simulink subsystem "SensorsRef"  (R2025a)
settings: Solver=VariableStepAuto  StartTime=0.0  StopTime=10.0  RelTol=1e-3
undefined symbols (not defined in the file): Accel_bIb, chi, Euler, gamma, gpsLLA, LaserAlt, Omeg_BIb, Pos_bIi, Q_i2b, SimIn, Vel_bIi, Vtot
libraries: libAxisTransformations x2, starslibMathOperations x2, starslibAxisTransformations x1
settings Model: Creator=drhill  LastModifiedBy=alhallmark
settings SolverCC: AlgebraicLoopSolver=TrustRegion
settings OptimizationCC: ReuseModelBlockBuffer=off
settings DebuggingCC: UnconnectedInputMsg=warning  UnconnectedOutputMsg=warning  UnconnectedLineMsg=warning
settings ModelReferenceCC: EnableRefExpFcnMdlSchedulingChecks=on
settings RTWCC: GPUComputeCapability=3.5  DLArmComputeVersion=19.05

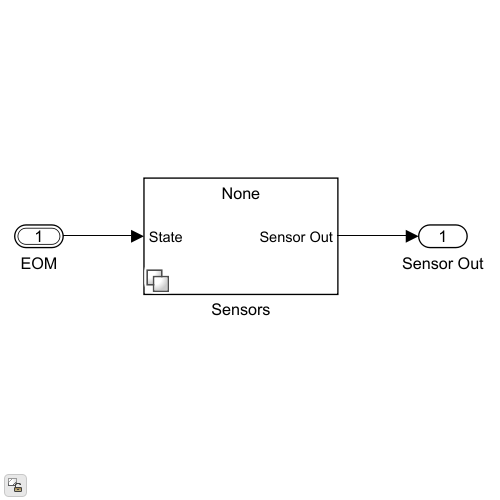
[thumbnail: Simulink's stored preview of the top-level diagram]
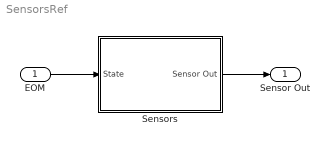
== system SensorsRef ==
  EOM : Inport  OutDataTypeStr=Bus: EomBus
  Sensors : Subsystem  Variant=on
  Sensor Out : Outport
  wires:
  Sensors/1(Sensor Out) -> Sensor Out/1
  EOM/1 -> Sensors/1(State)

== system SensorsRef/Sensors ==
  State : Inport  OutDataTypeStr=Bus: EomBus
  None : Subsystem  VariantControl=GVS_SENSOR_TYPE_NONE
  "ZOH " : Subsystem  VariantControl=GVS_SENSOR_TYPE_ZOH  mask{Sensor=SimIn.Sensor}
      mask prompts: Sensor "Sensor Data"
  Sensor Out : Outport  OutDataTypeStr=Bus: SensorBus  VectorParamsAs1DForOutWhenUnconnected=off

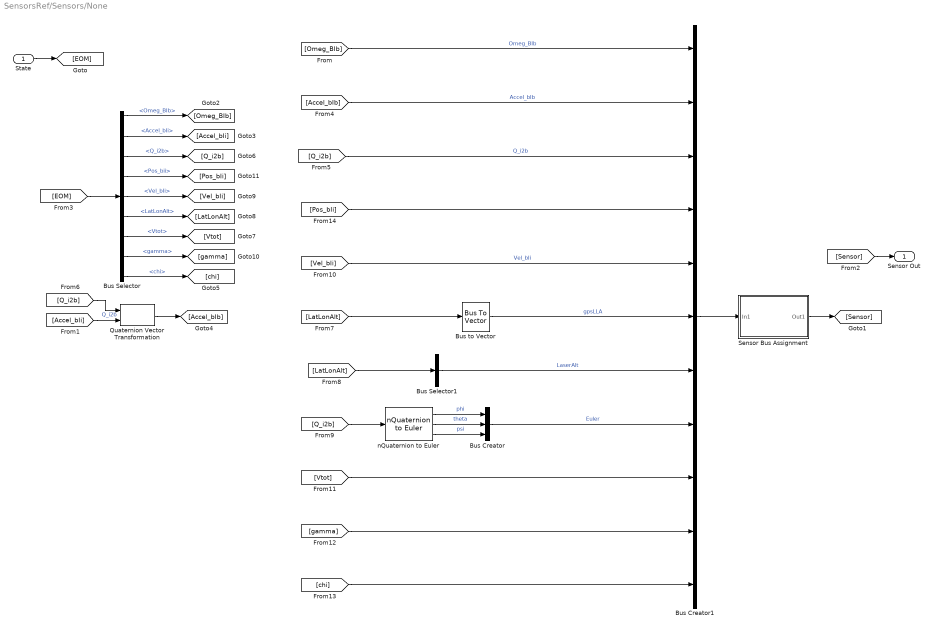
== system SensorsRef/Sensors/None ==
  State : Inport  OutDataTypeStr=Bus: EomBus
  Bus Creator : BusCreator  Inputs=3
  Bus Creator1 : BusCreator  Inputs=11
  Bus Selector : BusSelector  OutputSignals=InertialData.Omeg_BIb,InertialData.Accel_bIi,InertialData.Q_i2b,InertialData.Pos_bii,InertialData.Vel_bIi,WorldRelativeData.LatLonAlt,AirRelativeData.Vtot,AirRelativeData.gamma,AirRelativeData.chi
  Bus Selector1 : BusSelector  OutputSignals=AltGeod  OutputAsBus=on
  Bus to Vector : BusToVector
  Quaternion Vector Transformation : libAxisTransformations/Quaternion Vector Transformation  n=0
  Sensor Bus Assignment : Subsystem
  nQuaternion to Euler : libAxisTransformations/nQuaternion to Euler  n=1  RotOrd=ZYX
  Sensor Out : Outport  OutDataTypeStr=Bus: SensorBus  VectorParamsAs1DForOutWhenUnconnected=off
  wires:
  [Vel_bIi] -> Bus Creator1/5  "Vel_bIi"
  Bus Selector1/1 -> Bus Creator1/7  "LaserAlt"
  [Q_i2b] -> Bus Creator1/3  "Q_i2b"
  [Accel_bIb] -> Bus Creator1/2  "Accel_bIb"
  [Omeg_BIb] -> Bus Creator1/1  "Omeg_BIb"
  Bus Creator1/1 -> Sensor Bus Assignment/1(In1)
  State/1 -> [EOM]
  [EOM] -> Bus Selector/1
  Bus Selector/1 -> [Omeg_BIb]  "<Omeg_BIb>"
  Bus Selector/2 -> [Accel_bIi]  "<Accel_bIi>"
  Bus Selector/3 -> [Q_i2b]  "<Q_i2b>"
  Bus Selector/6 -> [LatLonAlt]  "<LatLonAlt>"
  [LatLonAlt] -> Bus Selector1/1
  Bus Selector/5 -> [Vel_bIi]  "<Vel_bIi>"
  Sensor Bus Assignment/1(Out1) -> [Sensor]
  [Sensor] -> Sensor Out/1
  [Q_i2b] -> Quaternion Vector Transformation/1  "Q_i2b"
  [Accel_bIi] -> Quaternion Vector Transformation/2
  Quaternion Vector Transformation/1 -> [Accel_bIb]
  Bus to Vector/1 -> Bus Creator1/6  "gpsLLA"
  [LatLonAlt] -> Bus to Vector/1
  [Q_i2b] -> nQuaternion to Euler/1
  nQuaternion to Euler/1 -> Bus Creator/1  "phi"
  nQuaternion to Euler/2 -> Bus Creator/2  "theta"
  nQuaternion to Euler/3 -> Bus Creator/3  "psi"
  Bus Creator/1 -> Bus Creator1/8  "Euler"
  Bus Selector/9 -> [chi]  "<chi>"
  Bus Selector/7 -> [Vtot]  "<Vtot>"
  Bus Selector/8 -> [gamma]  "<gamma>"
  [Vtot] -> Bus Creator1/9
  [gamma] -> Bus Creator1/10
  [chi] -> Bus Creator1/11
  Bus Selector/4 -> [Pos_bIi]  "<Pos_bii>"
  [Pos_bIi] -> Bus Creator1/4

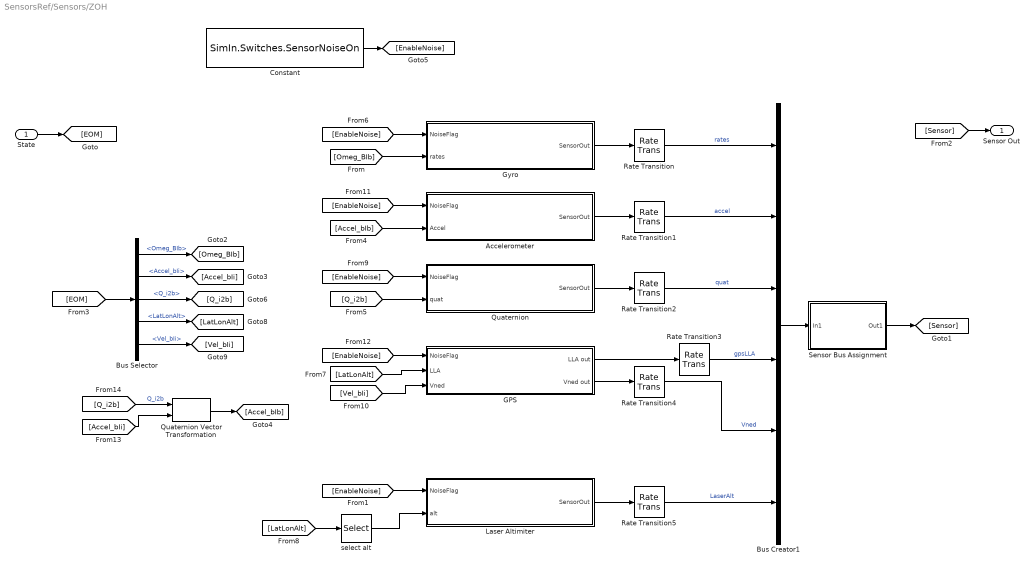
== system SensorsRef/Sensors/ZOH  ==
  State : Inport
  Accelerometer : Subsystem
  Bus Creator1 : BusCreator  Inputs=6
  Bus Selector : BusSelector  OutputSignals=Omeg_BIb,Accel_bIi,Q_i2b,LatLonAlt,Vel_bIi
  Constant : Constant  Value=SimIn.Switches.SensorNoiseOn
  GPS : Subsystem
  Gyro : Subsystem
  Laser Altimiter : Subsystem
  Quaternion : Subsystem
  Quaternion Vector Transformation : starslibAxisTransformations/Quaternion Vector Transformation  n=0
  Rate Transition{,1..5} (6 alike) : RateTransition  OutPortSampleTime=SimIn.Exec.FixedStep
  Sensor Bus Assignment : Subsystem
  select alt : Selector  InputPortWidth=3  IndexOptions=Index vector (dialog)  Indices=3  OutputSizes=1
  Sensor Out : Outport  VectorParamsAs1DForOutWhenUnconnected=off
  wires:
  [Sensor] -> Sensor Out/1
  GPS/2(Vned out) -> Rate Transition4/1
  [LatLonAlt] -> GPS/2(LLA)
  Bus Selector/4 -> [LatLonAlt]  "<LatLonAlt>"
  [Q_i2b] -> Quaternion/2(quat)
  Sensor Bus Assignment/1(Out1) -> [Sensor]
  Accelerometer/1(SensorOut) -> Rate Transition1/1
  [EnableNoise] -> Accelerometer/1(NoiseFlag)
  [EnableNoise] -> Gyro/1(NoiseFlag)
  [EnableNoise] -> Quaternion/1(NoiseFlag)
  [Accel_bIb] -> Accelerometer/2(Accel)
  [Omeg_BIb] -> Gyro/2(rates)
  [EOM] -> Bus Selector/1
  GPS/1(LLA out) -> Rate Transition3/1
  Quaternion/1(SensorOut) -> Rate Transition2/1
  Laser Altimiter/1(SensorOut) -> Rate Transition5/1
  [Vel_bIi] -> GPS/3(Vned)
  [EnableNoise] -> Laser Altimiter/1(NoiseFlag)
  State/1 -> [EOM]
  Bus Selector/5 -> [Vel_bIi]  "<Vel_bIi>"
  [LatLonAlt] -> select alt/1
  Gyro/1(SensorOut) -> Rate Transition/1
  Bus Creator1/1 -> Sensor Bus Assignment/1(In1)
  Constant/1 -> [EnableNoise]
  Bus Selector/1 -> [Omeg_BIb]  "<Omeg_BIb>"
  Bus Selector/2 -> [Accel_bIi]  "<Accel_bIi>"
  select alt/1 -> Laser Altimiter/2(alt)
  [EnableNoise] -> GPS/1(NoiseFlag)
  Bus Selector/3 -> [Q_i2b]  "<Q_i2b>"
  Rate Transition/1 -> Bus Creator1/1  "rates"
  Rate Transition1/1 -> Bus Creator1/2  "accel"
  Rate Transition2/1 -> Bus Creator1/3  "quat"
  Rate Transition3/1 -> Bus Creator1/4  "gpsLLA"
  Rate Transition4/1 -> Bus Creator1/5  "Vned"
  Rate Transition5/1 -> Bus Creator1/6  "LaserAlt"
  [Accel_bIi] -> Quaternion Vector Transformation/2
  [Q_i2b] -> Quaternion Vector Transformation/1  "Q_i2b"
  Quaternion Vector Transformation/1 -> [Accel_bIb]

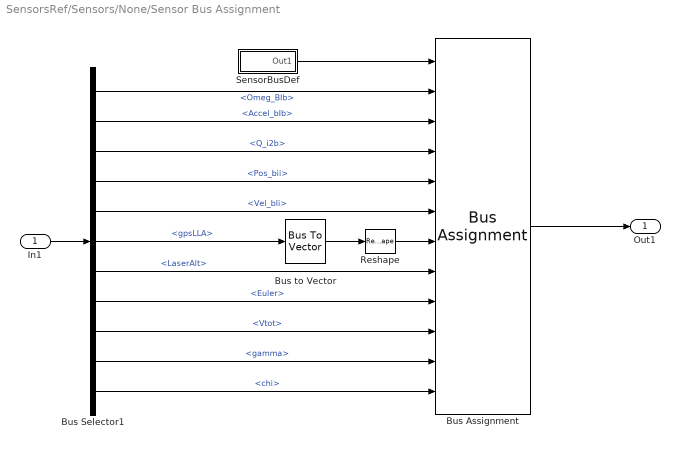
== system SensorsRef/Sensors/None/Sensor Bus Assignment ==
  In1 : Inport
  Bus Assignment : BusAssignment  AssignedSignals=Omeg_BIb,Accel_bIb,Q_i2b,Pos_bIi,Vel_bIi,gpsLLA,LaserAlt,Euler,Vtot,gamma,chi
  Bus Selector1 : BusSelector  OutputSignals=Omeg_BIb,Accel_bIb,Q_i2b,Pos_bii,Vel_bIi,gpsLLA,LaserAlt,Euler,Vtot,gamma,chi
  Bus to Vector : BusToVector
  Reshape : Reshape  OutputDimensionality=Column vector (2-D)
  SensorBusDef : Subsystem
  Out1 : Outport  VectorParamsAs1DForOutWhenUnconnected=off
  wires:
  Bus Assignment/1 -> Out1/1
  In1/1 -> Bus Selector1/1
  SensorBusDef/1(Out1) -> Bus Assignment/1
  Bus Selector1/7 -> Bus Assignment/8  "<LaserAlt>"
  Bus Selector1/1 -> Bus Assignment/2  "<Omeg_BIb>"
  Bus Selector1/6 -> Bus to Vector/1  "<gpsLLA>"
  Bus Selector1/3 -> Bus Assignment/4  "<Q_i2b>"
  Bus Selector1/5 -> Bus Assignment/6  "<Vel_bIi>"
  Bus Selector1/2 -> Bus Assignment/3  "<Accel_bIb>"
  Bus to Vector/1 -> Reshape/1
  Reshape/1 -> Bus Assignment/7
  Bus Selector1/8 -> Bus Assignment/9  "<Euler>"
  Bus Selector1/9 -> Bus Assignment/10  "<Vtot>"
  Bus Selector1/10 -> Bus Assignment/11  "<gamma>"
  Bus Selector1/11 -> Bus Assignment/12  "<chi>"
  Bus Selector1/4 -> Bus Assignment/5  "<Pos_bii>"

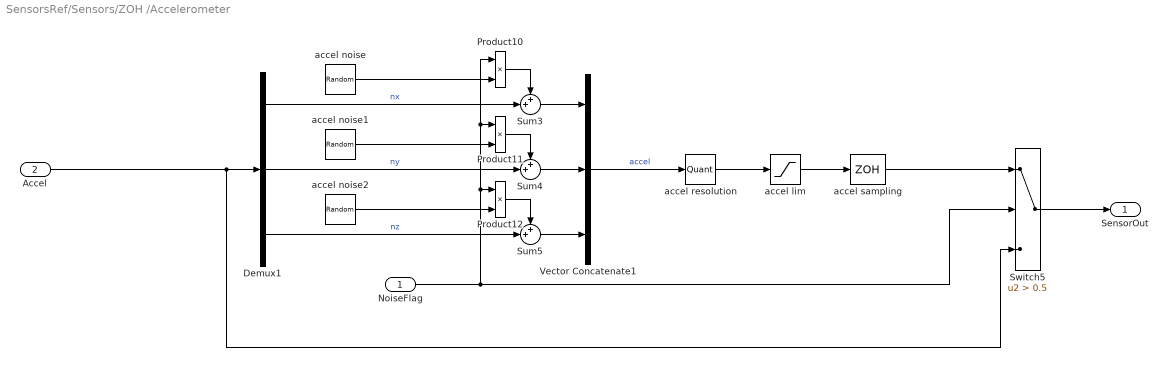
== system SensorsRef/Sensors/ZOH /Accelerometer ==
  NoiseFlag : Inport
  Accel : Inport  Port=2
  Demux1 : Demux  Outputs=3
  Product10 : Product
  Product11 : Product
  Product12 : Product
  Sum3 : Sum  Inputs=++|
  Sum4 : Sum  Inputs=++|
  Sum5 : Sum  Inputs=++|
  Switch5 : Switch  Criteria=u2 > Threshold  Threshold=0.5  SaturateOnIntegerOverflow=off  InputSameDT=off
  Vector Concatenate1 : Concatenate  NumInputs=3  Mode=Multidimensional array
  accel lim : Saturate  UpperLimit=Sensor.Accel.Lim  LowerLimit=-Sensor.Accel.Lim
  accel noise : RandomNumber  Mean=Sensor.Accel.X.bias  Variance=Sensor.Accel.X.var  Seed=Sensor.Accel.X.seed  SampleTime=Sensor.Accel.Tn
  accel noise1 : RandomNumber  Mean=Sensor.Accel.Y.bias  Variance=Sensor.Accel.Y.var  Seed=Sensor.Accel.Y.seed  SampleTime=Sensor.Accel.Tn
  accel noise2 : RandomNumber  Mean=Sensor.Accel.Y.bias  Variance=Sensor.Accel.Y.var  Seed=Sensor.Accel.Y.seed  SampleTime=Sensor.Accel.Tn
  accel resolution : Quantizer  QuantizationInterval=Sensor.Accel.Res
  accel sampling : ZeroOrderHold  SampleTime=Sensor.Accel.Ts
  SensorOut : Outport  VectorParamsAs1DForOutWhenUnconnected=off
  wires:
  Switch5/1 -> SensorOut/1
  accel sampling/1 -> Switch5/1
  Vector Concatenate1/1 -> accel resolution/1  "accel"
  accel lim/1 -> accel sampling/1
  accel resolution/1 -> accel lim/1
  Product11/1 -> Sum4/1
  NoiseFlag/1 -> Product12/1, Product11/1, Product10/1, Switch5/2
  Product10/1 -> Sum3/1
  accel noise/1 -> Product10/2
  accel noise1/1 -> Product11/2
  Accel/1 -> Demux1/1, Switch5/3
  accel noise2/1 -> Product12/2
  Product12/1 -> Sum5/1
  Sum4/1 -> Vector Concatenate1/2
  Sum5/1 -> Vector Concatenate1/3
  Sum3/1 -> Vector Concatenate1/1
  Demux1/3 -> Sum5/2  "nz"
  Demux1/1 -> Sum3/2  "nx"
  Demux1/2 -> Sum4/2  "ny"

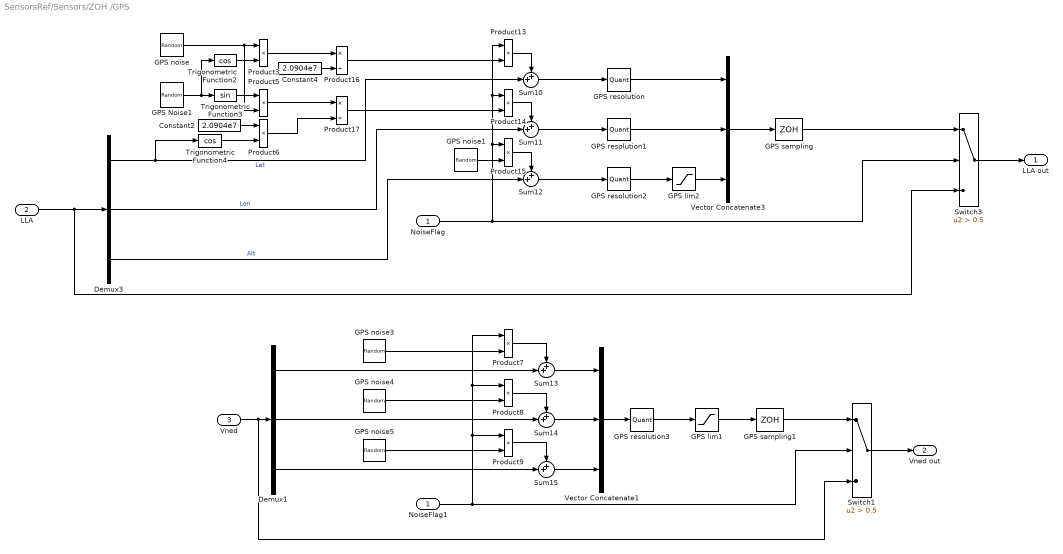
== system SensorsRef/Sensors/ZOH /GPS ==
  NoiseFlag : Inport
  LLA : Inport  Port=2
  Vned : Inport  Port=3
  Constant2 : Constant  Value=2.0904e7
  Constant4 : Constant  Value=2.0904e7
  Demux1 : Demux  Outputs=3
  Demux3 : Demux  Outputs=3
  GPS Noise1 : UniformRandomNumber  Minimum=Sensor.GPS.dir.min  Maximum=Sensor.GPS.dir.max  Seed=Sensor.GPS.dir.seed  SampleTime=Sensor.GPS.Tn
  GPS lim1 : Saturate  UpperLimit=Sensor.GPS.vel.Lim  LowerLimit=-Sensor.GPS.vel.Lim
  GPS lim2 : Saturate  UpperLimit=Sensor.GPS.alt.Lim  LowerLimit=0
  GPS noise : RandomNumber  Mean=Sensor.GPS.r.bias  Variance=Sensor.GPS.r.var  Seed=Sensor.GPS.r.seed  SampleTime=Sensor.GPS.Tn
  GPS noise1 : RandomNumber  Mean=Sensor.GPS.alt.bias  Variance=Sensor.GPS.alt.var  Seed=Sensor.GPS.alt.seed  SampleTime=Sensor.GPS.Tn
  GPS noise3 : RandomNumber  Mean=Sensor.GPS.Vn.bias  Variance=Sensor.GPS.Vn.var  Seed=Sensor.GPS.Vn.seed  SampleTime=Sensor.GPS.vel.Tn
  GPS noise4 : RandomNumber  Mean=Sensor.GPS.Ve.bias  Variance=Sensor.GPS.Ve.var  Seed=Sensor.GPS.Ve.seed  SampleTime=Sensor.GPS.vel.Tn
  GPS noise5 : RandomNumber  Mean=Sensor.GPS.Vd.bias  Variance=Sensor.GPS.Vd.var  Seed=Sensor.GPS.Vd.seed  SampleTime=Sensor.GPS.vel.Tn
  GPS resolution : Quantizer  QuantizationInterval=Sensor.GPS.Lat.Res
  GPS resolution1 : Quantizer  QuantizationInterval=Sensor.GPS.Lon.Res
  GPS resolution2 : Quantizer  QuantizationInterval=Sensor.GPS.alt.Res
  GPS resolution3 : Quantizer  QuantizationInterval=Sensor.GPS.vel.Res
  GPS sampling : ZeroOrderHold  SampleTime=Sensor.GPS.Ts
  GPS sampling1 : ZeroOrderHold  SampleTime=Sensor.GPS.Ts
  NoiseFlag1 : InportShadow
  Product{3,5..9,13..15} (9 alike) : Product
  Product16 : Product  Inputs=*/
  Product17 : Product  Inputs=*/
  Sum{10..15} (6 alike) : Sum  Inputs=++|
  Switch1 : Switch  Criteria=u2 > Threshold  Threshold=0.5  SaturateOnIntegerOverflow=off  InputSameDT=off
  Switch3 : Switch  Criteria=u2 > Threshold  Threshold=0.5  SaturateOnIntegerOverflow=off  InputSameDT=off
  Trigonometric Function2 : Trigonometry  Operator=cos
  Trigonometric Function3 : Trigonometry
  Trigonometric Function4 : Trigonometry  Operator=cos
  Vector Concatenate1 : Concatenate  NumInputs=3  Mode=Multidimensional array
  Vector Concatenate3 : Concatenate  NumInputs=3  Mode=Multidimensional array
  LLA out : Outport  VectorParamsAs1DForOutWhenUnconnected=off
  Vned out : Outport  Port=2  VectorParamsAs1DForOutWhenUnconnected=off
  wires:
  Switch1/1 -> Vned out/1
  NoiseFlag1/1 -> Switch1/2, Product9/1, Product8/1, Product7/1
  Vector Concatenate1/1 -> GPS resolution3/1
  GPS sampling1/1 -> Switch1/1
  GPS lim1/1 -> GPS sampling1/1
  GPS resolution3/1 -> GPS lim1/1
  Vned/1 -> Demux1/1, Switch1/3
  Product9/1 -> Sum15/1
  GPS noise5/1 -> Product9/2
  GPS noise3/1 -> Product7/2
  GPS noise4/1 -> Product8/2
  Product7/1 -> Sum13/1
  Product8/1 -> Sum14/1
  Sum15/1 -> Vector Concatenate1/3
  Sum13/1 -> Vector Concatenate1/1
  Demux1/2 -> Sum14/2
  Demux1/1 -> Sum13/2
  Sum14/1 -> Vector Concatenate1/2
  Demux1/3 -> Sum15/2
  Switch3/1 -> LLA out/1
  GPS sampling/1 -> Switch3/1
  GPS lim2/1 -> Vector Concatenate3/3
  GPS noise1/1 -> Product15/2
  Product17/1 -> Product14/2
  Product16/1 -> Product13/2
  Demux3/1 -> Trigonometric Function4/1, Sum10/2  "Lat"
  Product6/1 -> Product17/2
  Product5/1 -> Product17/1
  Product3/1 -> Product16/1
  Constant4/1 -> Product16/2
  Constant2/1 -> Product6/1
  Trigonometric Function4/1 -> Product6/2
  Trigonometric Function3/1 -> Product5/1
  GPS noise/1 -> Product3/1, Product5/2
  Trigonometric Function2/1 -> Product3/2
  GPS Noise1/1 -> Trigonometric Function3/1, Trigonometric Function2/1
  GPS resolution1/1 -> Vector Concatenate3/2
  GPS resolution/1 -> Vector Concatenate3/1
  Vector Concatenate3/1 -> GPS sampling/1
  Demux3/2 -> Sum11/2  "Lon"
  Demux3/3 -> Sum12/2  "Alt"
  LLA/1 -> Demux3/1, Switch3/3
  Product15/1 -> Sum12/1
  Product13/1 -> Sum10/1
  Sum10/1 -> GPS resolution/1
  Sum11/1 -> GPS resolution1/1
  Sum12/1 -> GPS resolution2/1
  Product14/1 -> Sum11/1
  NoiseFlag/1 -> Product15/1, Product14/1, Product13/1, Switch3/2
  GPS resolution2/1 -> GPS lim2/1

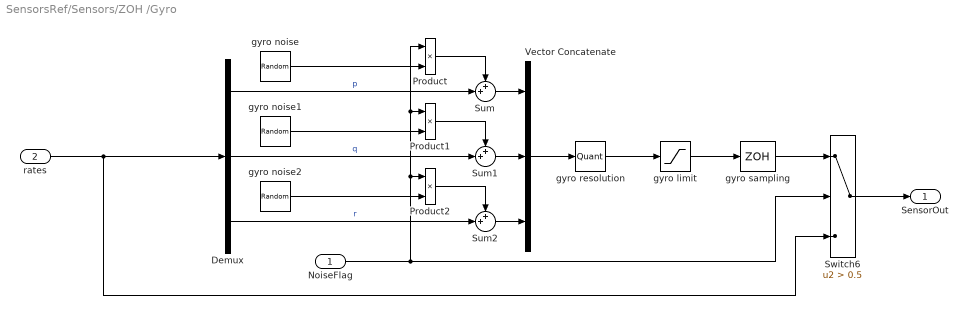
== system SensorsRef/Sensors/ZOH /Gyro ==
  NoiseFlag : Inport
  rates : Inport  Port=2
  Demux : Demux  Outputs=3
  Product : Product
  Product1 : Product
  Product2 : Product
  Sum : Sum  Inputs=++|
  Sum1 : Sum  Inputs=++|
  Sum2 : Sum  Inputs=++|
  Switch6 : Switch  Criteria=u2 > Threshold  Threshold=0.5  SaturateOnIntegerOverflow=off  InputSameDT=off
  Vector Concatenate : Concatenate  NumInputs=3  Mode=Multidimensional array
  gyro limit : Saturate  UpperLimit=Sensor.Gyro.Lim  LowerLimit=-Sensor.Gyro.Lim
  gyro noise : RandomNumber  Mean=Sensor.Gyro.X.bias  Variance=Sensor.Gyro.X.var  Seed=Sensor.Gyro.X.seed  SampleTime=Sensor.Gyro.Tn
  gyro noise1 : RandomNumber  Mean=SimIn.Sensor.Gyro.Y.bias  Variance=SimIn.Sensor.Gyro.Y.var  Seed=SimIn.Sensor.Gyro.Y.seed  SampleTime=SimIn.Sensor.Gyro.Tn  VectorParams1D=off
  gyro noise2 : RandomNumber  Mean=Sensor.Gyro.Z.bias  Variance=Sensor.Gyro.Z.var  Seed=Sensor.Gyro.Z.seed  SampleTime=Sensor.Gyro.Tn
  gyro resolution : Quantizer  QuantizationInterval=Sensor.Gyro.Res
  gyro sampling : ZeroOrderHold  SampleTime=Sensor.Gyro.Ts
  SensorOut : Outport  VectorParamsAs1DForOutWhenUnconnected=off
  wires:
  gyro limit/1 -> gyro sampling/1
  gyro resolution/1 -> gyro limit/1
  Demux/3 -> Sum2/2  "r"
  NoiseFlag/1 -> Product2/1, Product1/1, Product/1, Switch6/2
  Product2/1 -> Sum2/1
  gyro noise2/1 -> Product2/2
  Sum/1 -> Vector Concatenate/1
  Sum2/1 -> Vector Concatenate/3
  Vector Concatenate/1 -> gyro resolution/1
  Product/1 -> Sum/1
  gyro noise/1 -> Product/2
  Product1/1 -> Sum1/1
  gyro noise1/1 -> Product1/2
  Sum1/1 -> Vector Concatenate/2
  rates/1 -> Demux/1, Switch6/3
  Demux/2 -> Sum1/2  "q"
  Demux/1 -> Sum/2  "p"
  Switch6/1 -> SensorOut/1
  gyro sampling/1 -> Switch6/1

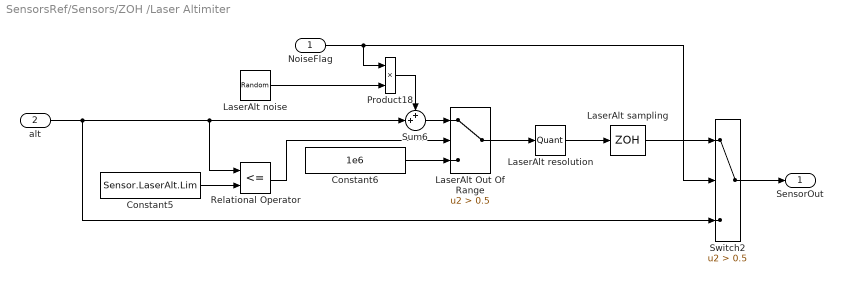
== system SensorsRef/Sensors/ZOH /Laser Altimiter ==
  NoiseFlag : Inport
  alt : Inport  Port=2
  Constant5 : Constant  Value=Sensor.LaserAlt.Lim
  Constant6 : Constant  Value=1e6
  LaserAlt Out Of Range : Switch  Criteria=u2 > Threshold  Threshold=0.5  SaturateOnIntegerOverflow=off  InputSameDT=off
  LaserAlt noise : RandomNumber  Mean=Sensor.LaserAlt.bias  Variance=Sensor.LaserAlt.var  Seed=Sensor.LaserAlt.seed  SampleTime=Sensor.LaserAlt.Tn
  LaserAlt resolution : Quantizer  QuantizationInterval=Sensor.LaserAlt.Res
  LaserAlt sampling : ZeroOrderHold  SampleTime=Sensor.LaserAlt.Ts
  Product18 : Product
  Relational Operator : RelationalOperator  Operator=<=  OutDataTypeStr=boolean  RndMeth=Simplest  InputSameDT=off
  Sum6 : Sum  Inputs=++|
  Switch2 : Switch  Criteria=u2 > Threshold  Threshold=0.5  SaturateOnIntegerOverflow=off  InputSameDT=off
  SensorOut : Outport  VectorParamsAs1DForOutWhenUnconnected=off
  wires:
  LaserAlt noise/1 -> Product18/2
  alt/1 -> Relational Operator/1, Sum6/2, Switch2/3
  Switch2/1 -> SensorOut/1
  NoiseFlag/1 -> Product18/1, Switch2/2
  LaserAlt sampling/1 -> Switch2/1
  LaserAlt Out Of Range/1 -> LaserAlt resolution/1
  Relational Operator/1 -> LaserAlt Out Of Range/2
  Constant6/1 -> LaserAlt Out Of Range/3
  Constant5/1 -> Relational Operator/2
  Product18/1 -> Sum6/1
  LaserAlt resolution/1 -> LaserAlt sampling/1
  Sum6/1 -> LaserAlt Out Of Range/1

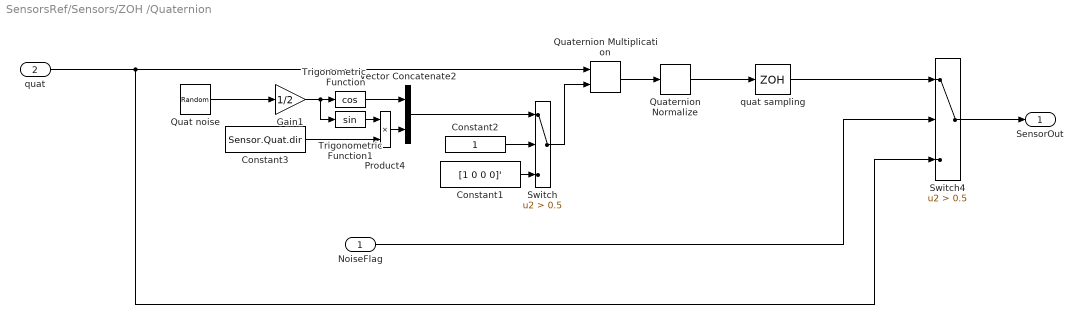
== system SensorsRef/Sensors/ZOH /Quaternion ==
  NoiseFlag : Inport
  quat : Inport  Port=2
  Constant1 : Constant  Value=[1 0 0 0]'
  Constant2 : Constant
  Constant3 : Constant  Value=Sensor.Quat.dir
  Gain1 : Gain  Gain=1/2
  Product4 : Product
  Quat noise : RandomNumber  Mean=Sensor.Quat.bias  Variance=Sensor.Quat.var  Seed=Sensor.Quat.seed  SampleTime=Sensor.Quat.Tn
  Quaternion Multiplication : starslibMathOperations/Quaternion Multiplication  n=0
  Quaternion Normalize : starslibMathOperations/Quaternion Normalize  n=0
  Switch : Switch  Criteria=u2 > Threshold  Threshold=0.5  SaturateOnIntegerOverflow=off  InputSameDT=off
  Switch4 : Switch  Criteria=u2 > Threshold  Threshold=0.5  SaturateOnIntegerOverflow=off  InputSameDT=off
  Trigonometric Function : Trigonometry  Operator=cos
  Trigonometric Function1 : Trigonometry
  Vector Concatenate2 : Concatenate  Mode=Multidimensional array
  quat sampling : ZeroOrderHold  SampleTime=Sensor.Quat.Ts
  SensorOut : Outport  VectorParamsAs1DForOutWhenUnconnected=off
  wires:
  quat sampling/1 -> Switch4/1
  Switch4/1 -> SensorOut/1
  quat/1 -> Quaternion Multiplication/1, Switch4/3
  Quat noise/1 -> Gain1/1
  Quaternion Multiplication/1 -> Quaternion Normalize/1
  Switch/1 -> Quaternion Multiplication/2
  Constant1/1 -> Switch/3
  Vector Concatenate2/1 -> Switch/1
  Trigonometric Function/1 -> Vector Concatenate2/1
  Product4/1 -> Vector Concatenate2/2
  Constant3/1 -> Product4/2
  Trigonometric Function1/1 -> Product4/1
  Gain1/1 -> Trigonometric Function/1, Trigonometric Function1/1
  NoiseFlag/1 -> Switch4/2
  Quaternion Normalize/1 -> quat sampling/1
  Constant2/1 -> Switch/2

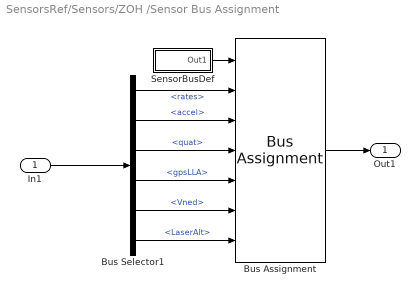
== system SensorsRef/Sensors/ZOH /Sensor Bus Assignment ==
  In1 : Inport
  Bus Assignment : BusAssignment  AssignedSignals=Omeg_BIb,Accel_bIb,Q_i2b,gpsLLA,Vel_bIi,LaserAlt
  Bus Selector1 : BusSelector  OutputSignals=rates,accel,quat,gpsLLA,Vned,LaserAlt
  SensorBusDef : Subsystem
  Out1 : Outport  VectorParamsAs1DForOutWhenUnconnected=off
  wires:
  Bus Assignment/1 -> Out1/1
  In1/1 -> Bus Selector1/1
  SensorBusDef/1(Out1) -> Bus Assignment/1
  Bus Selector1/6 -> Bus Assignment/7  "<LaserAlt>"
  Bus Selector1/1 -> Bus Assignment/2  "<rates>"
  Bus Selector1/4 -> Bus Assignment/5  "<gpsLLA>"
  Bus Selector1/3 -> Bus Assignment/4  "<quat>"
  Bus Selector1/5 -> Bus Assignment/6  "<Vned>"
  Bus Selector1/2 -> Bus Assignment/3  "<accel>"

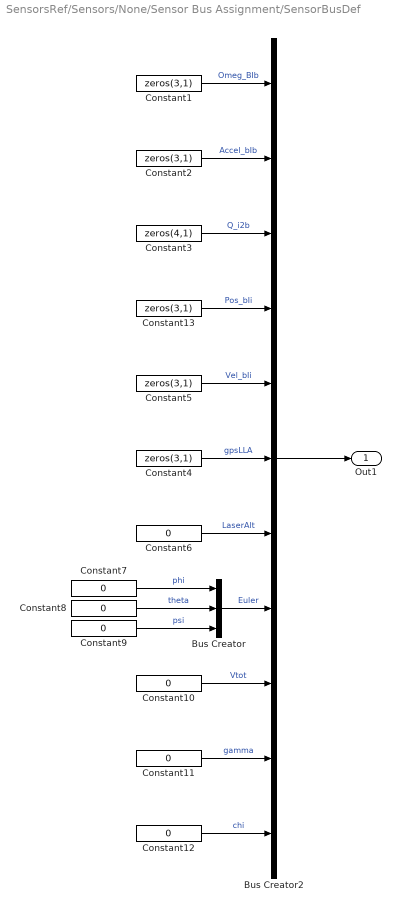
== system SensorsRef/Sensors/None/Sensor Bus Assignment/SensorBusDef ==
  Bus Creator : BusCreator  Inputs=3
  Bus Creator2 : BusCreator  Inputs=11  OutDataTypeStr=Bus: SensorBus
  Constant{1..2,4..5,13} (5 alike) : Constant  Value=zeros(3,1)  VectorParams1D=off
  Constant{6..12} (7 alike) : Constant  Value=0  VectorParams1D=off
  Constant3 : Constant  Value=zeros(4,1)  VectorParams1D=off
  Out1 : Outport  VectorParamsAs1DForOutWhenUnconnected=off
  wires:
  Constant4/1 -> Bus Creator2/6  "gpsLLA"
  Constant1/1 -> Bus Creator2/1  "Omeg_BIb"
  Constant2/1 -> Bus Creator2/2  "Accel_bIb"
  Constant3/1 -> Bus Creator2/3  "Q_i2b"
  Bus Creator2/1 -> Out1/1
  Constant6/1 -> Bus Creator2/7  "LaserAlt"
  Constant5/1 -> Bus Creator2/5  "Vel_bIi"
  Bus Creator/1 -> Bus Creator2/8  "Euler"
  Constant7/1 -> Bus Creator/1  "phi"
  Constant8/1 -> Bus Creator/2  "theta"
  Constant9/1 -> Bus Creator/3  "psi"
  Constant11/1 -> Bus Creator2/10  "gamma"
  Constant12/1 -> Bus Creator2/11  "chi"
  Constant10/1 -> Bus Creator2/9  "Vtot"
  Constant13/1 -> Bus Creator2/4  "Pos_bIi"

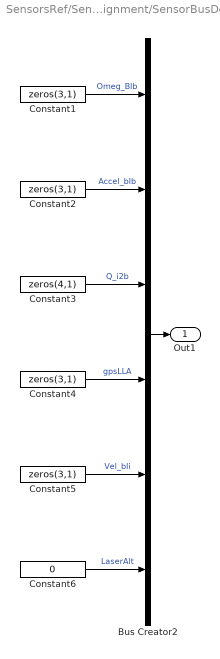
== system SensorsRef/Sensors/ZOH /Sensor Bus Assignment/SensorBusDef ==
  Bus Creator2 : BusCreator  Inputs=6  OutDataTypeStr=Bus: SensorBus
  Constant{1..2,4..5} (4 alike) : Constant  Value=zeros(3,1)  VectorParams1D=off
  Constant3 : Constant  Value=zeros(4,1)  VectorParams1D=off
  Constant6 : Constant  Value=0  VectorParams1D=off
  Out1 : Outport  VectorParamsAs1DForOutWhenUnconnected=off
  wires:
  Constant4/1 -> Bus Creator2/4  "gpsLLA"
  Constant1/1 -> Bus Creator2/1  "Omeg_BIb"
  Constant2/1 -> Bus Creator2/2  "Accel_bIb"
  Constant3/1 -> Bus Creator2/3  "Q_i2b"
  Bus Creator2/1 -> Out1/1
  Constant6/1 -> Bus Creator2/6  "LaserAlt"
  Constant5/1 -> Bus Creator2/5  "Vel_bIi"
